simulink library "sm_car_lib"  (R2026a)
settings: Solver=VariableStepAuto
undefined symbols (not defined in the file or in its folder): acc_theta, accel_ramp_rate, circ_out, clr_upr, Control, hp1, hp2, hp3, hp_in_f_ua, hp_in_r_ua, hp_la_out, hp_ua_out, Init, Newton, opc_upr, radius_upr, Raphson, RDF_Rough_Road, rhs_hp, Scene, ShaftF, ShaftR, Vehicle, Visual, X, Y, Z
libraries: sm_lib x115, $bdroot x92, nesl_utility x36, simulink x17, fl_lib x6, sharedtransformsys x3, Brakes_Elements x2, Multibody_Parts_Lib x2, Aero_Coefficients x1, Body_Axle2 x1, BodyGeometry_Sedan x1, Brakes_Axle2 x1
(part 6 of 6)

== system sm_car_lib/Inputs/Control Bus Axle3/SuspF ==
  Bus Creator{1..5,7} (6 alike) : BusCreator  Inputs=1
  Constant : Constant
  SuspA1 : Outport  VectorParamsAs1DForOutWhenUnconnected=off
  SuspA2 : Outport  Port=2  VectorParamsAs1DForOutWhenUnconnected=off
  SuspA3 : Outport  Port=3  VectorParamsAs1DForOutWhenUnconnected=off
  wires:
  Bus Creator3/1 -> SuspA2/1  "SuspA2"
  Bus Creator1/1 -> SuspA1/1  "SuspA1"
  Bus Creator5/1 -> SuspA3/1  "SuspA3"
  Bus Creator7/1 -> Bus Creator1/1  "Steer"
  Bus Creator4/1 -> Bus Creator3/1  "Steer"
  Bus Creator2/1 -> Bus Creator5/1  "Steer"
  Constant/1 -> Bus Creator7/1, Bus Creator2/1, Bus Creator4/1  "aSteerWheel"

== system sm_car_lib/Inputs/Control Bus Axle3/Torque Input ==
  Bus Creator : BusCreator  Inputs=2
  Front Torque Enable : Gain
  Rear Torque Enable : Gain
  Torque Front : Subsystem  mask{on_time=1, off_time=10, torque_value=torque_fa}
      mask prompts: on_time "On Time (s)"; off_time "Off Time (s)"; torque_value "Torque Value (N*m)"
      mask TypeOptions on_time: Step On/Time
      mask TypeOptions off_time: Step Off/Time
      mask TypeOptions torque_value: Step Height/Gain
  Torque Rear : Subsystem  mask{on_time=1, off_time=10, torque_value=torque_ra}
      mask prompts: on_time "On Time (s)"; off_time "Off Time (s)"; torque_value "Torque Value (N*m)"
      mask TypeOptions on_time: Step On/Time
      mask TypeOptions off_time: Step Off/Time
      mask TypeOptions torque_value: Step Height/Gain
  Driveline : Outport  VectorParamsAs1DForOutWhenUnconnected=off
  wires:
  Torque Rear/1(MMotorRDemand) -> Rear Torque Enable/1
  Bus Creator/1 -> Driveline/1  "Driveline"
  Front Torque Enable/1 -> Bus Creator/1  "MMotorA1Demand"
  Rear Torque Enable/1 -> Bus Creator/2  "MMotorA2Demand"
  Torque Front/1(MMotorRDemand) -> Front Torque Enable/1

== system sm_car_lib/Inputs/DrvBus/Accel ==
  Step : Step  Time=brake_on_time  FinalValue=[1 1 1 1]  SampleTime=0  ZeroCross=off
  Brk : Outport  VectorParamsAs1DForOutWhenUnconnected=off
  wires:
  Step/1 -> Brk/1  "rBrakePedal"

== system sm_car_lib/Inputs/DrvBus/Brake ==
  Step : Step  Time=brake_on_time  SampleTime=0  ZeroCross=off
  Brk : Outport  VectorParamsAs1DForOutWhenUnconnected=off
  wires:
  Step/1 -> Brk/1  "rBrakePedal"

== system sm_car_lib/Inputs/DrvBus/Steer Input ==
  Constant : Constant  Value=popup_steer_input
  Lane Change : simulink/Sources/Repeating Sequence  rep_seq_t=[0 10 10.5 11.5 12 13 13.5 20]  rep_seq_y=[0 0 1 1 -1 -1 0 0]*5*pi/180
  Multiport Switch : MultiPortSwitch  Inputs=4  SaturateOnIntegerOverflow=off  InputSameDT=off
  No Steer : Constant  Value=0
  Sequence : simulink/Sources/Repeating Sequence  rep_seq_t=[0 1 2 3 4 5]  rep_seq_y=[0 0 -1 1 0 0]*5*pi/180
  Signal Specification : SignalSpecification  Unit=rad
  Step : Step  Time=5  FinalValue=5*pi/180  SampleTime=0  ZeroCross=off
      settings: AttributesFormatString=%<After> @ %<Time> sec
  DrvBus : Outport  VectorParamsAs1DForOutWhenUnconnected=off
  wires:
  Sequence/1 -> Multiport Switch/4  "aStrWhlF"
  Constant/1 -> Multiport Switch/1
  Step/1 -> Multiport Switch/3  "aStrWhlF"
  No Steer/1 -> Multiport Switch/2
  Signal Specification/1 -> DrvBus/1  "aSteerWheel"
  Lane Change/1 -> Multiport Switch/5  "aStrWhlF"
  Multiport Switch/1 -> Signal Specification/1

== system sm_car_lib/Inputs/DrvBus/Torque Input ==
  Torque Front : Subsystem  mask{on_time=1, off_time=10, rPedalValue=rPedalValue}
      mask prompts: on_time "On Time (s)"; off_time "Off Time (s)"; rPedalValue "Torque Value (N*m)"
      mask TypeOptions on_time: Step On/Time
      mask TypeOptions off_time: Step Off/Time
      mask TypeOptions rPedalValue: Gain/Gain
  rAccelPedal : Outport  VectorParamsAs1DForOutWhenUnconnected=off
  wires:
  Torque Front/1(rAccelPedal) -> rAccelPedal/1  "rAccelPedal"

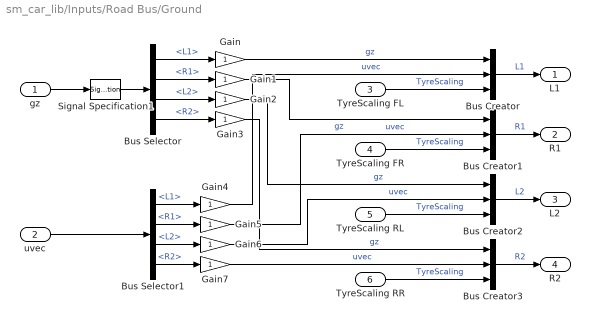
== system sm_car_lib/Inputs/Road Bus/Ground ==
  gz : Inport
  uvec : Inport  Port=2
  TyreScaling FL : Inport  Port=3
  TyreScaling FR : Inport  Port=4
  TyreScaling RL : Inport  Port=5
  TyreScaling RR : Inport  Port=6
  Bus Creator{,1..3} (4 alike) : BusCreator  Inputs=3
  Bus Selector : BusSelector  OutputSignals=L1,R1,L2,R2
  Bus Selector1 : BusSelector  OutputSignals=L1,R1,L2,R2
  Gain{,1..7} (8 alike) : Gain
  Signal Specification1 : SignalSpecification  Unit=m
  L1 : Outport  VectorParamsAs1DForOutWhenUnconnected=off
  R1 : Outport  Port=2  VectorParamsAs1DForOutWhenUnconnected=off
  L2 : Outport  Port=3  VectorParamsAs1DForOutWhenUnconnected=off
  R2 : Outport  Port=4  VectorParamsAs1DForOutWhenUnconnected=off
  wires:
  Gain7/1 -> Bus Creator3/2  "uvec"
  Gain6/1 -> Bus Creator2/2  "uvec"
  Gain5/1 -> Bus Creator1/2  "uvec"
  Gain4/1 -> Bus Creator/2  "uvec"
  Bus Selector1/4 -> Gain7/1  "<R2>"
  Bus Selector1/3 -> Gain6/1  "<L2>"
  Bus Selector1/2 -> Gain5/1  "<R1>"
  Bus Selector1/1 -> Gain4/1  "<L1>"
  uvec/1 -> Bus Selector1/1
  Bus Selector/4 -> Gain3/1  "<R2>"
  Bus Selector/3 -> Gain2/1  "<L2>"
  Bus Selector/2 -> Gain1/1  "<R1>"
  Gain/1 -> Bus Creator/1  "gz"
  Bus Selector/1 -> Gain/1  "<L1>"
  TyreScaling RR/1 -> Bus Creator3/3  "TyreScaling"
  TyreScaling RL/1 -> Bus Creator2/3  "TyreScaling"
  TyreScaling FR/1 -> Bus Creator1/3  "TyreScaling"
  Gain2/1 -> Bus Creator2/1  "gz"
  Signal Specification1/1 -> Bus Selector/1
  Bus Creator2/1 -> L2/1  "L2"
  Gain3/1 -> Bus Creator3/1  "gz"
  gz/1 -> Signal Specification1/1
  Bus Creator3/1 -> R2/1  "R2"
  TyreScaling FL/1 -> Bus Creator/3  "TyreScaling"
  Gain1/1 -> Bus Creator1/1  "gz"
  Bus Creator1/1 -> R1/1  "R1"
  Bus Creator/1 -> L1/1  "L1"

== system sm_car_lib/Inputs/Road Bus/None ==
  Bus Creator : BusCreator  Inputs=4
  Bus Creator1 : BusCreator  Inputs=4
  Constant : Constant  Value=[0 0 0 0]
  Constant{1..4} (4 alike) : Constant  Value=[0 0 1]
  Demux2 : Demux
  Signal Specification1 : SignalSpecification  Unit=m
  gz : Outport  VectorParamsAs1DForOutWhenUnconnected=off
  uvec : Outport  Port=2  VectorParamsAs1DForOutWhenUnconnected=off
  wires:
  Bus Creator/1 -> uvec/1  "uvec"
  Constant4/1 -> Bus Creator/4  "R2"
  Constant1/1 -> Bus Creator/1  "L1"
  Constant2/1 -> Bus Creator/2  "R1"
  Constant3/1 -> Bus Creator/3  "L2"
  Demux2/3 -> Bus Creator1/3  "L2"
  Demux2/4 -> Bus Creator1/4  "R2"
  Demux2/2 -> Bus Creator1/2  "R1"
  Bus Creator1/1 -> gz/1  "gz"
  Signal Specification1/1 -> Demux2/1
  Demux2/1 -> Bus Creator1/1  "L1"
  Constant/1 -> Signal Specification1/1

== system sm_car_lib/Outputs/VehBus/Brakes ==
  Bus Creator1 : BusCreator  Inputs=4
  Subsystem : Subsystem
  Subsystem1 : $bdroot/Outputs/VehBus/Brakes/Subsystem  SystemSampleTime=-1  VariantActivationTime=update diagram  EmptyChoice=off  PassThrough=off  PassThroughVariantControl=(default)  EmptyChoiceVariantControl=(default)  AllowFlexibleInterface=on  Latency=0  AutoFrameSizeCalculation=off
  Subsystem2 : $bdroot/Outputs/VehBus/Brakes/Subsystem  SystemSampleTime=-1  VariantActivationTime=update diagram  EmptyChoice=off  PassThrough=off  PassThroughVariantControl=(default)  EmptyChoiceVariantControl=(default)  AllowFlexibleInterface=on  Latency=0  AutoFrameSizeCalculation=off
  Subsystem3 : $bdroot/Outputs/VehBus/Brakes/Subsystem  SystemSampleTime=-1  VariantActivationTime=update diagram  EmptyChoice=off  PassThrough=off  PassThroughVariantControl=(default)  EmptyChoiceVariantControl=(default)  AllowFlexibleInterface=on  Latency=0  AutoFrameSizeCalculation=off
  Brakes : Outport  VectorParamsAs1DForOutWhenUnconnected=off
  wires:
  Bus Creator1/1 -> Brakes/1
  Subsystem/1(Whl) -> Bus Creator1/1  "L1"
  Subsystem1/1 -> Bus Creator1/2  "R1"
  Subsystem2/1 -> Bus Creator1/3  "L2"
  Subsystem3/1 -> Bus Creator1/4  "R2"

== system sm_car_lib/Outputs/VehBus/Subsystem ==
  Aero : Subsystem
  Body{,1..4} (5 alike) : $bdroot/Sensors/Body Sensor  offset_body_sensor=Vehicle.Chassis.Body.sCG.Value
  Bus Creator1 : BusCreator  Inputs=4
  Bus Creator2 : BusCreator  Inputs=10
  Bus Creator3 : BusCreator  Inputs=2
  Constant8 : Constant
  Constant9 : Constant
  Damper : Subsystem
  Source : Subsystem
  Spring : Subsystem
  Subsystem1 : $bdroot/Outputs/VehBus/Subsystem/Source  SystemSampleTime=-1  VariantActivationTime=update diagram  EmptyChoice=off  PassThrough=off  PassThroughVariantControl=(default)  EmptyChoiceVariantControl=(default)  AllowFlexibleInterface=on  Latency=0  AutoFrameSizeCalculation=off
  Subsystem2 : $bdroot/Outputs/VehBus/Subsystem/Source  SystemSampleTime=-1  VariantActivationTime=update diagram  EmptyChoice=off  PassThrough=off  PassThroughVariantControl=(default)  EmptyChoiceVariantControl=(default)  AllowFlexibleInterface=on  Latency=0  AutoFrameSizeCalculation=off
  Subsystem3 : $bdroot/Outputs/VehBus/Subsystem/Source  SystemSampleTime=-1  VariantActivationTime=update diagram  EmptyChoice=off  PassThrough=off  PassThroughVariantControl=(default)  EmptyChoiceVariantControl=(default)  AllowFlexibleInterface=on  Latency=0  AutoFrameSizeCalculation=off
  B : PMIOPort  Side=Left
  Chassis : Outport  VectorParamsAs1DForOutWhenUnconnected=off
  wires:
  Subsystem1/1 -> Bus Creator2/4  "WhlR1"
  Damper/1(Damper) -> Bus Creator2/2  "Damper"
  Bus Creator2/1 -> Chassis/1  "Chassis"
  Subsystem2/1 -> Bus Creator2/5  "WhlL2"
  Subsystem3/1 -> Bus Creator2/6  "WhlR2"
  Constant8/1 -> Bus Creator2/8  "SuspA1"
  Constant9/1 -> Bus Creator2/9  "SuspA2"
  Source/1(Whl) -> Bus Creator2/3  "WhlL1"
  Spring/1(Spring) -> Bus Creator2/1  "Spring"
  Aero/1(Aero) -> Bus Creator2/7  "Aero"
  Bus Creator3/1 -> Bus Creator2/10  "Body"
  Body/1 -> Bus Creator3/1  "CG"
  Body1/1 -> Bus Creator1/1  "FL"
  Body2/1 -> Bus Creator1/2  "FR"
  Body3/1 -> Bus Creator1/3  "RL"
  Body4/1 -> Bus Creator1/4  "RR"
  Bus Creator1/1 -> Bus Creator3/2  "Passengers"
  connections:
  Body/LConn1 -- Body4/LConn1 -- Body3/LConn1 -- Body2/LConn1 -- Body1/LConn1 -- B/RConn1

== system sm_car_lib/Sensors/Body Sensor/Roll Pitch ==
  R : Inport
  Calculate aPitch : Subsystem
  Calculate aRoll : Subsystem
  "Flip sign for -x axis " : Gain  Gain=-1
  Select x axis : Selector  NumberOfDimensions=2  InputPortWidth=2  IndexOptions=Index vector (dialog),Index vector (dialog)  Indices=[1 2 3],1  OutputSizes=1,1
  Select y axis : Selector  NumberOfDimensions=2  InputPortWidth=2  IndexOptions=Index vector (dialog),Index vector (dialog)  Indices=[1 2 3],2  OutputSizes=1,1
  Transfer Fcn : TransferFcn  Numerator=[1 0]  Denominator=[0.01 1]
  Transfer Fcn1 : TransferFcn  Numerator=[1 0]  Denominator=[0.01 1]
  aRoll : Outport  VectorParamsAs1DForOutWhenUnconnected=off
  aPitch : Outport  Port=2  VectorParamsAs1DForOutWhenUnconnected=off
  nRoll : Outport  Port=3  VectorParamsAs1DForOutWhenUnconnected=off
  nPitch : Outport  Port=4  VectorParamsAs1DForOutWhenUnconnected=off
  wires:
  Calculate aPitch/1(Angle) -> "Flip sign for -x axis "/1
  Select x axis/1 -> Calculate aPitch/2(uvec)
  R/1 -> Select y axis/1, Select x axis/1
  Select y axis/1 -> Calculate aRoll/1(uvec)
  "Flip sign for -x axis "/1 -> aPitch/1, Transfer Fcn1/1
  Calculate aRoll/1(Angle) -> Transfer Fcn/1, aRoll/1, Calculate aPitch/1(Roll Angle)
  Transfer Fcn/1 -> nRoll/1
  Transfer Fcn1/1 -> nPitch/1

== system sm_car_lib/Suspensions/Wheel Measurements/Calculate Camber ==
  uvec spin axis : Inport
  Demux : Demux  Outputs=3
  Mux : Mux  Inputs=2
  Trigonometric Function1 : Trigonometry  Operator=atan2
  magnitude : Fcn  Expr=sqrt(u(1)*u(1)+u(2)*u(2))
  Camber : Outport  VectorParamsAs1DForOutWhenUnconnected=off
  wires:
  Demux/1 -> Mux/1
  uvec spin axis/1 -> Demux/1
  Trigonometric Function1/1 -> Camber/1
  Demux/3 -> Trigonometric Function1/1
  Mux/1 -> magnitude/1
  magnitude/1 -> Trigonometric Function1/2
  Demux/2 -> Mux/2

== system sm_car_lib/Suspensions/Wheel Measurements/Calculate Camber Z Axis ==
  uvec spin axis : Inport
  Demux : Demux  Outputs=3
  Mux : Mux  Inputs=2
  Trigonometric Function1 : Trigonometry  Operator=atan2
  magnitude : Fcn  Expr=sqrt(u(1)*u(1)+u(2)*u(2))
  Camber : Outport  VectorParamsAs1DForOutWhenUnconnected=off
  wires:
  Demux/2 -> Mux/2
  magnitude/1 -> Trigonometric Function1/2
  Mux/1 -> magnitude/1
  Demux/3 -> Trigonometric Function1/1
  Trigonometric Function1/1 -> Camber/1
  uvec spin axis/1 -> Demux/1
  Demux/1 -> Mux/1

== system sm_car_lib/Suspensions/Wheel Measurements/Calculate Toe ==
  uvec spin axis : Inport
  Demux : Demux  Outputs=3
  Gain : Gain
  Gain1 : Gain
  Terminator : Terminator
  Trigonometric Function1 : Trigonometry  Operator=atan2
  Toe : Outport  VectorParamsAs1DForOutWhenUnconnected=off
  wires:
  Demux/2 -> Gain1/1
  uvec spin axis/1 -> Demux/1
  Demux/1 -> Gain/1
  Demux/3 -> Terminator/1
  Gain/1 -> Trigonometric Function1/1
  Gain1/1 -> Trigonometric Function1/2
  Trigonometric Function1/1 -> Toe/1

== system sm_car_lib/Suspensions/Wheel Measurements/Calculate Toe X Axis ==
  uvec spin axis : Inport
  Demux : Demux  Outputs=3
  Gain : Gain
  Gain1 : Gain
  Terminator : Terminator
  Trigonometric Function1 : Trigonometry  Operator=atan2
  Toe : Outport  VectorParamsAs1DForOutWhenUnconnected=off
  wires:
  Trigonometric Function1/1 -> Toe/1
  Gain1/1 -> Trigonometric Function1/2
  Gain/1 -> Trigonometric Function1/1
  Demux/3 -> Terminator/1
  Demux/1 -> Gain/1
  uvec spin axis/1 -> Demux/1
  Demux/2 -> Gain1/1

== system sm_car_lib/Utilities/Q to Z-Y-X Extrinsic/Subsystem ==
  q : Inport
  r11 : Inport  Port=2
  r12 : Inport  Port=3
  r21 : Inport  Port=4
  In4 : Inport  Port=5
  r32 : Inport  Port=6
  Subsystem : Subsystem
  Terminator : Terminator
  Trigonometric Function1 : Trigonometry  Operator=atan2
  Trigonometric Function3 : Trigonometry  Operator=atan2
  Vector Concatenate : Concatenate  NumInputs=3
  trigFcn : Trigonometry  Operator=asin
  R1,R2,R3 : Outport  VectorParamsAs1DForOutWhenUnconnected=off
  wires:
  Vector Concatenate/1 -> R1,R2,R3/1
  r12/1 -> Trigonometric Function1/2
  r21/1 -> Subsystem/1(In)
  r11/1 -> Trigonometric Function1/1
  r32/1 -> Trigonometric Function3/2
  trigFcn/1 -> Vector Concatenate/2  "r2"
  q/1 -> Terminator/1
  Subsystem/1(Out) -> trigFcn/1
  Trigonometric Function3/1 -> Vector Concatenate/3  "r3"
  Trigonometric Function1/1 -> Vector Concatenate/1  "r1"
  In4/1 -> Trigonometric Function3/1

== system sm_car_lib/Utilities/Q to Z-Y-X Extrinsic/Subsystem1 ==
  q : Inport  Unit=1
  Demux : Demux
  Mux : Mux
  Product{,1..3} (4 alike) : Product  Inputs=*/
  Subsystem : Subsystem
  qnorm : Outport  Unit=1  VectorParamsAs1DForOutWhenUnconnected=off
  wires:
  Product2/1 -> Mux/3
  Demux/2 -> Product1/1
  q/1 -> Subsystem/1(In1), Demux/1
  Demux/4 -> Product3/1
  Demux/3 -> Product2/1
  Product/1 -> Mux/1
  Mux/1 -> qnorm/1
  Subsystem/1(Out1) -> Product3/2, Product2/2, Product/2, Product1/2
  Demux/1 -> Product/1
  Product3/1 -> Mux/4
  Product1/1 -> Mux/2

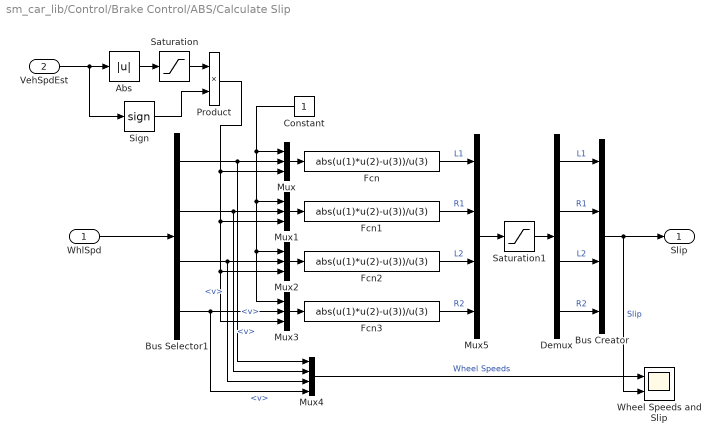
== system sm_car_lib/Control/Brake Control/ABS/Calculate Slip ==
  WhlSpd : Inport
  VehSpdEst : Inport  Port=2
  Abs : Abs  ZeroCross=off  SaturateOnIntegerOverflow=off
  Bus Creator : BusCreator  Inputs=4
  Bus Selector1 : BusSelector  OutputSignals=L1.v,R1.v,L2.v,R2.v
  Constant : Constant
  Demux : Demux
  Fcn{,1..3} (4 alike) : Fcn  Expr=abs(u(1)*u(2)-u(3))/u(3)
  Mux{,1..3} (4 alike) : Mux  Inputs=3
  Mux4 : Mux
  Mux5 : Mux
  Product : Product
  Saturation : Saturate  UpperLimit=inf  LowerLimit=eps  ZeroCross=off
  Saturation1 : Saturate  UpperLimit=1  LowerLimit=0
  Sign : Signum  ZeroCross=off
  Wheel Speeds and Slip : Scope  NumInputPorts=2
      settings: ActiveDisplayYMinimum=-11.64241  ActiveDisplayYMaximum=114.01232  DataLoggingVariableName=ScopeData2
  Slip : Outport  VectorParamsAs1DForOutWhenUnconnected=off
  wires:
  WhlSpd/1 -> Bus Selector1/1
  Bus Selector1/2 -> Mux4/2, Mux1/2  "<v>"
  Bus Selector1/4 -> Mux4/4, Mux3/2  "<v>"
  Bus Selector1/1 -> Mux4/1, Mux/2  "<v>"
  Bus Selector1/3 -> Mux4/3, Mux2/2  "<v>"
  Constant/1 -> Mux/1, Mux1/1, Mux3/1, Mux2/1
  VehSpdEst/1 -> Sign/1, Abs/1
  Demux/1 -> Bus Creator/1  "L1"
  Demux/2 -> Bus Creator/2  "R1"
  Demux/3 -> Bus Creator/3  "L2"
  Demux/4 -> Bus Creator/4  "R2"
  Bus Creator/1 -> Wheel Speeds and Slip/2, Slip/1  "Slip"
  Product/1 -> Mux3/3, Mux2/3, Mux1/3, Mux/3
  Abs/1 -> Saturation/1
  Saturation/1 -> Product/1
  Sign/1 -> Product/2
  Mux/1 -> Fcn/1
  Mux1/1 -> Fcn1/1
  Mux2/1 -> Fcn2/1
  Mux3/1 -> Fcn3/1
  Mux4/1 -> Wheel Speeds and Slip/1  "Wheel Speeds"
  Mux5/1 -> Saturation1/1
  Saturation1/1 -> Demux/1
  Fcn/1 -> Mux5/1  "L1"
  Fcn1/1 -> Mux5/2  "R1"
  Fcn2/1 -> Mux5/3  "L2"
  Fcn3/1 -> Mux5/4  "R2"

== system sm_car_lib/Control/Brake Control/ABS/Sensor ==
  Body : Inport
  WhlSpd : Inport  Port=2
  Bus Creator{,3..5} (4 alike) : BusCreator  Inputs=1
  Bus Creator6 : BusCreator  Inputs=5
  Bus Selector : BusSelector  OutputSignals=vx,vy  OutputAsBus=on
  Bus Selector4 : BusSelector  OutputSignals=WhlL1.n,WhlR1.n,WhlL2.n,WhlR2.n,WhlL2.qxyz
  Gain : Gain  Gain=3.6*abs_tire_radiusF
  Gain1 : Gain  Gain=3.6*abs_tire_radiusF
  Gain2 : Gain  Gain=3.6*abs_tire_radiusR
  Gain3 : Gain  Gain=3.6*abs_tire_radiusR
  Gain4 : Gain  Gain=3.6
  Terminator1 : Terminator  Commented=on
  Vel in xy plane : Fcn  Expr=sqrt(u(1)^2+u(2)^2)
  missing tooth : Subsystem  Commented=on
  GroundSpd : Outport  VectorParamsAs1DForOutWhenUnconnected=off
  wires:
  Gain1/1 -> Bus Creator3/1  "v"
  missing tooth/1(Out1) -> Terminator1/1  "v"
  Gain2/1 -> Bus Creator4/1  "v"
  Bus Selector4/5 -> missing tooth/2(<qxyz>)  "<qxyz>"
  Bus Creator5/1 -> Bus Creator6/5  "R2"
  Gain3/1 -> Bus Creator5/1  "v"
  Bus Creator/1 -> Bus Creator6/2  "L1"
  Bus Selector4/2 -> Gain1/1  "<n>"
  Bus Creator4/1 -> Bus Creator6/4  "L2"
  Bus Selector4/3 -> Gain2/1, missing tooth/1(<omega>)  "<n>"
  Gain/1 -> Bus Creator/1  "v"
  Body/1 -> Bus Selector/1
  Bus Creator3/1 -> Bus Creator6/3  "R1"
  Gain4/1 -> Bus Creator6/1  "v"
  Bus Selector4/1 -> Gain/1  "<n>"
  Bus Selector4/4 -> Gain3/1  "<n>"
  WhlSpd/1 -> Bus Selector4/1
  Bus Creator6/1 -> GroundSpd/1
  Vel in xy plane/1 -> Gain4/1  "speed"
  Bus Selector/1 -> Vel in xy plane/1

== system sm_car_lib/Control/Brake Control/ABS/Vehicle Speed ==
  Sensors : Inport
  Bus Selector : BusSelector  OutputSignals=v
  vSpdEst : Outport  VectorParamsAs1DForOutWhenUnconnected=off
  wires:
  Sensors/1 -> Bus Selector/1
  Bus Selector/1 -> vSpdEst/1  "<v>"

== system sm_car_lib/Control/Valve Control/Categorize Surface/Count Apply Pulses ==
  In1 : Inport
  Trigger : TriggerPort  VariantControl=Variant
  Constant : Constant  Value=0
  Memory : Memory  InheritSampleTime=on
  Pulse Increment : Constant
  Sum : Sum  Inputs=|++
  Switch : Switch  Criteria=u2 > Threshold  Threshold=0.5  ZeroCross=off  SaturateOnIntegerOverflow=off  InputSameDT=off
  Apply Pulses : Outport  VectorParamsAs1DForOutWhenUnconnected=off
  wires:
  Pulse Increment/1 -> Sum/2
  Sum/1 -> Switch/3, Apply Pulses/1
  Memory/1 -> Sum/1
  In1/1 -> Switch/2
  Constant/1 -> Switch/1
  Switch/1 -> Memory/1

== system sm_car_lib/Control/Valve Control/Categorize Surface/Total Apply Pulses This Cycle ==
  In1 : Inport
  Trigger : TriggerPort  VariantControl=Variant
  Total Pulses : Outport  VectorParamsAs1DForOutWhenUnconnected=off
  wires:
  In1/1 -> Total Pulses/1

== system sm_car_lib/Environment/CarWorldConfig/Mechanism Configuration/Constant Gravity ==
  MechanismConfiguration : sm_lib/Utilities/Mechanism Configuration  UniformGravity=Constant  GravityVector=GravityVector  GravityVectorUnits=m/s^2  LinearizationDelta=0.001  JointModeTransitionNonlinearIterations=2
  C : PMIOPort  Side=Right
  connections:
  MechanismConfiguration/RConn1 -- C/RConn1

== system sm_car_lib/Environment/CarWorldConfig/Mechanism Configuration/Variable GravityXY ==
  Constant : Constant  Value=acc_theta
  Constant1 : Constant  Value=GravityVector(3)
  MechanismConfiguration : sm_lib/Utilities/Mechanism Configuration  UniformGravity=TimeVarying  GravityVector=[0 0 -9.80665]  GravityVectorUnits=m/s^2  LinearizationDelta=0.001  JointModeTransitionNonlinearIterations=2
  Mux : Mux  Inputs=3
  Product : Product
  Product1 : Product
  Ramp1 : simulink/Sources/Ramp  slope=accel_ramp_rate  start=2  InitialOutput=0
  Scope : Scope
      settings: ActiveDisplayYMinimum=-1.12718  ActiveDisplayYMaximum=10.14459
  Simulink-PS Converter : nesl_utility/Simulink-PS Converter  PhysicalDomain=network_engine_domain  SubClassName=ps_input  LeftPortType=input  RightPortType=output  PseudoPeriodic=off  Frequencies=[]  NoiseDistribution=none  NoiseParameters=[]  Unit=m/s^2  AffineConversion=off  FilteringAndDerivatives=provide  SimscapeFilterOrder=1  InputFilterTimeConstant=0.001  UdotUserProvided=0
  Sin : Trigonometry
  Sin1 : Trigonometry  Operator=cos
  C : PMIOPort  Side=Right
  wires:
  Ramp1/1 -> Product/2, Product1/2, Scope/1  "accel_xy"
  Product1/1 -> Mux/1
  Constant1/1 -> Mux/3
  Sin/1 -> Product/1
  Mux/1 -> Simulink-PS Converter/1
  Sin1/1 -> Product1/1
  Constant/1 -> Sin/1, Sin1/1
  Product/1 -> Mux/2
  connections:
  MechanismConfiguration/LConn1 -- Simulink-PS Converter/RConn1
  MechanismConfiguration/RConn1 -- C/RConn1

== system sm_car_lib/Inputs/Control Bus/Torque Input/Torque Front ==
  Gain : Gain
  Rate Limiter : RateLimiter  RisingSlewLimit=300  FallingSlewLimit=-300  SampleTimeMode=inherited
  Step Height : Gain  Gain=torque_value
  Step Off : Step  Time=off_time  FinalValue=-1  SampleTime=0  ZeroCross=off
  Step On : Step  Time=on_time  SampleTime=0  ZeroCross=off
  Sum : Sum  Inputs=|++
  MMotorRDemand : Outport  VectorParamsAs1DForOutWhenUnconnected=off
  wires:
  Gain/1 -> MMotorRDemand/1  "MMotorRDemand"
  Step Off/1 -> Sum/2
  Sum/1 -> Step Height/1
  Step On/1 -> Sum/1
  Rate Limiter/1 -> Gain/1
  Step Height/1 -> Rate Limiter/1

== system sm_car_lib/Inputs/Control Bus/Torque Input/Torque Rear ==
  Gain : Gain
  Rate Limiter : RateLimiter  RisingSlewLimit=300  FallingSlewLimit=-300  SampleTimeMode=inherited
  Step Height : Gain  Gain=torque_value
  Step Off : Step  Time=off_time  FinalValue=-1  SampleTime=0  ZeroCross=off
  Step On : Step  Time=on_time  SampleTime=0  ZeroCross=off
  Sum : Sum  Inputs=|++
  MMotorRDemand : Outport  VectorParamsAs1DForOutWhenUnconnected=off
  wires:
  Step Height/1 -> Rate Limiter/1
  Rate Limiter/1 -> Gain/1
  Step On/1 -> Sum/1
  Sum/1 -> Step Height/1
  Step Off/1 -> Sum/2
  Gain/1 -> MMotorRDemand/1  "MMotorRDemand"

== system sm_car_lib/Inputs/Control Bus Axle3/Torque Input/Torque Front ==
  Gain : Gain
  Rate Limiter : RateLimiter  RisingSlewLimit=300  FallingSlewLimit=-300  SampleTimeMode=inherited
  Step Height : Gain  Gain=torque_value
  Step Off : Step  Time=off_time  FinalValue=-1  SampleTime=0  ZeroCross=off
  Step On : Step  Time=on_time  SampleTime=0  ZeroCross=off
  Sum : Sum  Inputs=|++
  MMotorRDemand : Outport  VectorParamsAs1DForOutWhenUnconnected=off
  wires:
  Step Height/1 -> Rate Limiter/1
  Rate Limiter/1 -> Gain/1
  Step On/1 -> Sum/1
  Sum/1 -> Step Height/1
  Step Off/1 -> Sum/2
  Gain/1 -> MMotorRDemand/1  "MMotorRDemand"

== system sm_car_lib/Inputs/Control Bus Axle3/Torque Input/Torque Rear ==
  Gain : Gain
  Rate Limiter : RateLimiter  RisingSlewLimit=300  FallingSlewLimit=-300  SampleTimeMode=inherited
  Step Height : Gain  Gain=torque_value
  Step Off : Step  Time=off_time  FinalValue=-1  SampleTime=0  ZeroCross=off
  Step On : Step  Time=on_time  SampleTime=0  ZeroCross=off
  Sum : Sum  Inputs=|++
  MMotorRDemand : Outport  VectorParamsAs1DForOutWhenUnconnected=off
  wires:
  Gain/1 -> MMotorRDemand/1  "MMotorRDemand"
  Step Off/1 -> Sum/2
  Sum/1 -> Step Height/1
  Step On/1 -> Sum/1
  Rate Limiter/1 -> Gain/1
  Step Height/1 -> Rate Limiter/1

== system sm_car_lib/Inputs/DrvBus/Torque Input/Torque Front ==
  Gain : Gain  Gain=rPedalValue
  Step Off : Step  Time=off_time  FinalValue=-1  SampleTime=0  ZeroCross=off
  Step On : Step  Time=on_time  SampleTime=0  ZeroCross=off
  Sum : Sum  Inputs=|++
  rAccelPedal : Outport  VectorParamsAs1DForOutWhenUnconnected=off
  wires:
  Sum/1 -> Gain/1
  Step Off/1 -> Sum/2
  Step On/1 -> Sum/1
  Gain/1 -> rAccelPedal/1  "rAccelPedal"

== system sm_car_lib/Outputs/VehBus/Brakes/Subsystem ==
  Bus Creator : BusCreator  Inputs=2
  Constant : Constant
  Constant1 : Constant
  Whl : Outport  VectorParamsAs1DForOutWhenUnconnected=off
  wires:
  Constant/1 -> Bus Creator/1  "trq"
  Bus Creator/1 -> Whl/1
  Constant1/1 -> Bus Creator/2  "p"

== system sm_car_lib/Outputs/VehBus/Subsystem/Aero ==
  Bus Creator : BusCreator  Inputs=2
  Constant1 : Constant
  Constant3 : Constant
  Aero : Outport  VectorParamsAs1DForOutWhenUnconnected=off
  wires:
  Constant3/1 -> Bus Creator/1  "Fx"
  Constant1/1 -> Bus Creator/2  "Fz"
  Bus Creator/1 -> Aero/1  "Aero"

== system sm_car_lib/Outputs/VehBus/Subsystem/Damper ==
  Bus Creator5 : BusCreator  Inputs=4
  Subsystem : Subsystem
  Subsystem1 : $bdroot/Outputs/VehBus/Subsystem/Damper/Subsystem  SystemSampleTime=-1  VariantActivationTime=update diagram  EmptyChoice=off  PassThrough=off  PassThroughVariantControl=(default)  EmptyChoiceVariantControl=(default)  AllowFlexibleInterface=on  Latency=0  AutoFrameSizeCalculation=off
  Subsystem2 : $bdroot/Outputs/VehBus/Subsystem/Damper/Subsystem  SystemSampleTime=-1  VariantActivationTime=update diagram  EmptyChoice=off  PassThrough=off  PassThroughVariantControl=(default)  EmptyChoiceVariantControl=(default)  AllowFlexibleInterface=on  Latency=0  AutoFrameSizeCalculation=off
  Subsystem3 : $bdroot/Outputs/VehBus/Subsystem/Damper/Subsystem  SystemSampleTime=-1  VariantActivationTime=update diagram  EmptyChoice=off  PassThrough=off  PassThroughVariantControl=(default)  EmptyChoiceVariantControl=(default)  AllowFlexibleInterface=on  Latency=0  AutoFrameSizeCalculation=off
  Damper : Outport  VectorParamsAs1DForOutWhenUnconnected=off
  wires:
  Subsystem3/1 -> Bus Creator5/4  "R2"
  Subsystem1/1 -> Bus Creator5/2  "R1"
  Bus Creator5/1 -> Damper/1  "Damper"
  Subsystem2/1 -> Bus Creator5/3  "L2"
  Subsystem/1(out) -> Bus Creator5/1  "L1"

== system sm_car_lib/Outputs/VehBus/Subsystem/Source ==
  Bus Creator : BusCreator  Inputs=15
  Constant1 : Constant  Value=[1 1 1]
  Constant{2..5,7..15} (13 alike) : Constant
  Constant6 : Constant  Value=[1 1 1]
  Whl : Outport  VectorParamsAs1DForOutWhenUnconnected=off
  wires:
  Constant11/1 -> Bus Creator/3  "n"
  Constant12/1 -> Bus Creator/4  "Fx"
  Constant1/1 -> Bus Creator/2  "xyz"
  Constant6/1 -> Bus Creator/1  "qxyz"
  Bus Creator/1 -> Whl/1
  Constant2/1 -> Bus Creator/5  "Fy"
  Constant3/1 -> Bus Creator/6  "Fz"
  Constant4/1 -> Bus Creator/7  "Mx"
  Constant5/1 -> Bus Creator/8  "My"
  Constant7/1 -> Bus Creator/9  "Mz"
  Constant8/1 -> Bus Creator/10  "rSlip"
  Constant9/1 -> Bus Creator/11  "aSlip"
  Constant10/1 -> Bus Creator/12  "aCamber"
  Constant13/1 -> Bus Creator/13  "vx"
  Constant14/1 -> Bus Creator/14  "rMuX"
  Constant15/1 -> Bus Creator/15  "rMuY"

== system sm_car_lib/Outputs/VehBus/Subsystem/Spring ==
  Bus Creator5 : BusCreator  Inputs=4
  Source : Subsystem
  Subsystem1 : $bdroot/Outputs/VehBus/Subsystem/Spring/Source  SystemSampleTime=-1  VariantActivationTime=update diagram  EmptyChoice=off  PassThrough=off  PassThroughVariantControl=(default)  EmptyChoiceVariantControl=(default)  AllowFlexibleInterface=on  Latency=0  AutoFrameSizeCalculation=off
  Subsystem2 : $bdroot/Outputs/VehBus/Subsystem/Spring/Source  SystemSampleTime=-1  VariantActivationTime=update diagram  EmptyChoice=off  PassThrough=off  PassThroughVariantControl=(default)  EmptyChoiceVariantControl=(default)  AllowFlexibleInterface=on  Latency=0  AutoFrameSizeCalculation=off
  Subsystem3 : $bdroot/Outputs/VehBus/Subsystem/Spring/Source  SystemSampleTime=-1  VariantActivationTime=update diagram  EmptyChoice=off  PassThrough=off  PassThroughVariantControl=(default)  EmptyChoiceVariantControl=(default)  AllowFlexibleInterface=on  Latency=0  AutoFrameSizeCalculation=off
  Spring : Outport  VectorParamsAs1DForOutWhenUnconnected=off
  wires:
  Bus Creator5/1 -> Spring/1  "Spring"
  Subsystem1/1 -> Bus Creator5/2  "R1"
  Subsystem2/1 -> Bus Creator5/3  "L2"
  Subsystem3/1 -> Bus Creator5/4  "R2"
  Source/1(out) -> Bus Creator5/1  "L1"

== system sm_car_lib/Sensors/Body Sensor/Roll Pitch/Calculate aPitch ==
  Roll Angle : Inport
  uvec : Inport  Port=2
  Asin : Trigonometry  Operator=asin
  Cos : Trigonometry  Operator=cos
  Divide : Product  Inputs=*/
  Divide1 : Product  Inputs=*/
  Selector : Selector  InputPortWidth=3  IndexOptions=Index vector (dialog)  Indices=[3]  OutputSizes=1
  magnitude : Fcn  Expr=sqrt(u(1)*u(1)+u(2)*u(2)+u(3)*u(3))
  Angle : Outport  VectorParamsAs1DForOutWhenUnconnected=off
  wires:
  Divide1/1 -> Asin/1
  uvec/1 -> magnitude/1, Selector/1
  magnitude/1 -> Divide1/2
  Selector/1 -> Divide/1
  Roll Angle/1 -> Cos/1
  Asin/1 -> Angle/1
  Divide/1 -> Divide1/1
  Cos/1 -> Divide/2

== system sm_car_lib/Sensors/Body Sensor/Roll Pitch/Calculate aRoll ==
  uvec : Inport
  Demux : Demux  Outputs=3
  Mux : Mux  Inputs=2
  Trigonometric Function1 : Trigonometry  Operator=atan2
  magnitude : Fcn  Expr=sqrt(u(1)*u(1)+u(2)*u(2))
  Angle : Outport  VectorParamsAs1DForOutWhenUnconnected=off
  wires:
  Demux/2 -> Mux/2
  magnitude/1 -> Trigonometric Function1/2
  Mux/1 -> magnitude/1
  Demux/3 -> Trigonometric Function1/1
  Trigonometric Function1/1 -> Angle/1
  uvec/1 -> Demux/1
  Demux/1 -> Mux/1

== system sm_car_lib/Utilities/Q to Z-Y-X Extrinsic/Subsystem/Subsystem ==
  In : Inport
  If : If  IfExpression=u1 > 1  ElseIfExpressions=u1 < -1
  If Action Subsystem : sharedtransformsys/Protect asincos input/If Action Subsystem  SystemSampleTime=-1  VariantActivationTime=update diagram  EmptyChoice=off  PassThrough=off  PassThroughVariantControl=(default)  EmptyChoiceVariantControl=(default)  AllowFlexibleInterface=on  Latency=0  AutoFrameSizeCalculation=off
  If Action Subsystem1 : sharedtransformsys/Protect asincos input/If Action Subsystem1  SystemSampleTime=-1  VariantActivationTime=update diagram  EmptyChoice=off  PassThrough=off  PassThroughVariantControl=(default)  EmptyChoiceVariantControl=(default)  AllowFlexibleInterface=on  Latency=0  AutoFrameSizeCalculation=off
  If Action Subsystem2 : sharedtransformsys/Protect asincos input/If Action Subsystem2  SystemSampleTime=-1  VariantActivationTime=update diagram  EmptyChoice=off  PassThrough=off  PassThroughVariantControl=(default)  EmptyChoiceVariantControl=(default)  AllowFlexibleInterface=on  Latency=0  AutoFrameSizeCalculation=off
  Merge : Merge  Inputs=3
  Out : Outport  VectorParamsAs1DForOutWhenUnconnected=off
  wires:
  If Action Subsystem1/1 -> Merge/2
  If/1 -> If Action Subsystem/Action
  In/1 -> If/1, If Action Subsystem2/1
  If/3 -> If Action Subsystem2/Action
  If Action Subsystem2/1 -> Merge/3
  If/2 -> If Action Subsystem1/Action
  If Action Subsystem/1 -> Merge/1
  Merge/1 -> Out/1

== system sm_car_lib/Utilities/Q to Z-Y-X Extrinsic/Subsystem1/Subsystem ==
  In1 : Inport
  Demux : Demux
  Product{,1..3} (4 alike) : Product
  Sum : Sum  Inputs=4
  sqrt : Sqrt  AlgorithmType=Newton-Raphson
  Out1 : Outport  VectorParamsAs1DForOutWhenUnconnected=off
  wires:
  Sum/1 -> sqrt/1
  sqrt/1 -> Out1/1
  In1/1 -> Demux/1
  Product3/1 -> Sum/4
  Demux/2 -> Product1/1, Product1/2
  Demux/1 -> Product/1, Product/2
  Product2/1 -> Sum/3
  Product/1 -> Sum/1
  Demux/3 -> Product2/1, Product2/2
  Product1/1 -> Sum/2
  Demux/4 -> Product3/1, Product3/2

== system sm_car_lib/Control/Brake Control/ABS/Sensor/missing tooth ==
  <omega> : Inport
  <qxyz> : Inport  Port=2
  Constant : Constant  Value=2*pi
  Constant1 : Constant  Value=0.5
  Constant2 : Constant
  Product : Product
  Rem : Math  Operator=rem  SignedPower=on
  Scope : Scope  NumInputPorts=5
      settings: ActiveDisplayYMinimum=-41.32335  ActiveDisplayYMaximum=259.55855  DataLoggingVariableName=ScopeData2
  Selector : Selector  InputPortWidth=3  IndexOptions=Index vector (dialog)  Indices=[2]  OutputSizes=1
  Subsystem : Subsystem  mask{int_limit_upper=25/48*2*pi, int_limit_lower=22/48*2*pi}
      mask prompts: int_limit_upper "Upper Limit"; int_limit_lower "Lower Limit"
      mask TypeOptions int_limit_upper: Upper Limit/Value
      mask TypeOptions int_limit_lower: Lower Limit/Value
  Switch : Switch  Criteria=u2 > Threshold  Threshold=0.5  SaturateOnIntegerOverflow=off  InputSameDT=off
  Out1 : Outport  VectorParamsAs1DForOutWhenUnconnected=off
  wires:
  <qxyz>/1 -> Scope/1, Selector/1
  Constant/1 -> Rem/2
  Rem/1 -> Scope/3, Subsystem/1(u)
  Selector/1 -> Scope/2, Rem/1
  Subsystem/1(y) -> Scope/4, Switch/2
  Switch/1 -> Scope/5, Product/2
  Constant1/1 -> Switch/1
  Constant2/1 -> Switch/3
  <omega>/1 -> Product/1
  Product/1 -> Out1/1

== system sm_car_lib/Outputs/VehBus/Subsystem/Damper/Subsystem ==
  Bus Creator : BusCreator  Inputs=4
  Constant{1..4} (4 alike) : Constant
  out : Outport  VectorParamsAs1DForOutWhenUnconnected=off
  wires:
  Constant2/1 -> Bus Creator/3  "xDamper"
  Bus Creator/1 -> out/1
  Constant3/1 -> Bus Creator/4  "vDamper"
  Constant1/1 -> Bus Creator/2  "FBumpstop"
  Constant4/1 -> Bus Creator/1  "FDamper"

== system sm_car_lib/Outputs/VehBus/Subsystem/Spring/Source ==
  Bus Creator : BusCreator  Inputs=2
  Constant1 : Constant
  Constant4 : Constant
  out : Outport  VectorParamsAs1DForOutWhenUnconnected=off
  wires:
  Constant1/1 -> Bus Creator/2  "FSpring"
  Constant4/1 -> Bus Creator/1  "xSpring"
  Bus Creator/1 -> out/1

== system sm_car_lib/Control/Brake Control/ABS/Sensor/missing tooth/Subsystem ==
  u : Inport
  AND : Logic  AllPortsSameDT=off  OutDataTypeStr=boolean
  FixPt Data Type Duplicate : DataTypeDuplicate  DisableCoverage=on  NumInputPorts=3
  Lower Limit : Constant  DisableCoverage=on  Value=int_limit_lower  OutDataTypeStr=Inherit: Inherit via back propagation
  Lower Test : RelationalOperator  DisableCoverage=on  Operator=<=  OutDataTypeStr=boolean  InputSameDT=off
  Upper Limit : Constant  DisableCoverage=on  Value=int_limit_upper  OutDataTypeStr=Inherit: Inherit via back propagation
  Upper Test : RelationalOperator  DisableCoverage=on  Operator=<=  OutDataTypeStr=boolean  InputSameDT=off
  y : Outport  VectorParamsAs1DForOutWhenUnconnected=off
  wires:
  Lower Limit/1 -> FixPt Data Type Duplicate/2, Lower Test/1
  Upper Limit/1 -> FixPt Data Type Duplicate/3, Upper Test/2
  u/1 -> Upper Test/1, Lower Test/2, FixPt Data Type Duplicate/1
  AND/1 -> y/1
  Upper Test/1 -> AND/2
  Lower Test/1 -> AND/1

== stateflow chart sm_car_lib/Control/Valve Control/Logic ==
  state Inactive
    entry:
    Mod_State = 1;
    Mod_Dur = 10;
  state Initial_Release
    entry:
    Mod_State = 2;
    Mod_Dur = 10;
  state Initial_Apply
    entry:
    Mod_State = 1;
    Mod_Dur = 6;
  state Release
    entry:
    Mod_State = 2;
    Mod_Dur = 6;
  state Apply
    entry:
    Mod_State = 1;
    Mod_Dur = 2;
  state Hold
    entry:
    Mod_State = 0;
    Mod_Dur = 6;
  (default) -> Inactive
  Apply -> Inactive [order 2] : [vSpdEst <0.1]
  Release -> Inactive [order 2] : [vSpdEst <0.1]
  Inactive -> Initial_Release : [Slip>0.5]
  Initial_Release -> Initial_Apply : [Slip<0.1]
  Release -> Initial_Apply [order 1] : [Slip <0.05]
  Initial_Apply -> Hold [order 2] : [Slip>0.1]
  Initial_Apply -> Apply [order 1] : [after(10,msec)]
  Hold -> Release [order 2] : [Slip > 0.25]
  Hold -> Apply [order 1] : [after(40,msec)]
  Apply -> Hold [order 1] : [Slip > 0.1]
  data: Slip input; Mod_State output; Mod_Dur output; vSpdEst input
